simulink model "B_SISO_Simulink"  (R2019a)
settings: Solver=VariableStepAuto  StartTime=0.0  StopTime=50  RelTol=1e-3
values from neighbouring files (symbols this model uses):
  A = [yv (yp+aa0) (yr - 1) (g*cos(tt0)/u0); l_lv l_lp l_lr 0; n_lv n_lp n_lr 0; 0 1 tan(tt0) 0]    [A_Anel_Aberto.m]    (also in B_SISO.m; C_D_LQR_e_Sensores.m = [yv (yp+aa0) (yr - 1) (g*cos(tt0)/u0) 0; l_lv l_lp l_lr 0 0;)
  B = [Yda Ydr ; Lda Ldr ; Nda Ndr ; 0 0]    [A_Anel_Aberto.m]    (also in B_SISO.m; C_D_LQR_e_Sensores.m = [Yda Ydr ; Lda Ldr ; Nda Ndr ; 0 0; 0 0])
  C = [1 0 0 0 ; 0 1 0 0 ; 0 0 1 0 ; 0 0 0 1]    [A_Anel_Aberto.m]    (also in B_SISO.m; C_D_LQR_e_Sensores.m = [1 0 0 0 0; 0 1 0 0 0; 0 0 1 0 0; 0 0 0 1 0; 0 0 0 0 1])
  D = [0 0; 0 0; 0 0; 0 0]    [A_Anel_Aberto.m]    (also in B_SISO.m; C_D_LQR_e_Sensores.m = [0 0; 0 0; 0 0; 0 0; 0 0])
  deg = pi/180    (= 0.0174532777778)    [A_Anel_Aberto.m]    (also in B_SISO.m; C_D_LQR_e_Sensores.m)
  kp = 4.7    [B_SISO.m]
  kr = 1.83    [B_SISO.m]
settings Model: Creator=Antonio Oliveira  LastModifiedBy=Antonio Oliveira

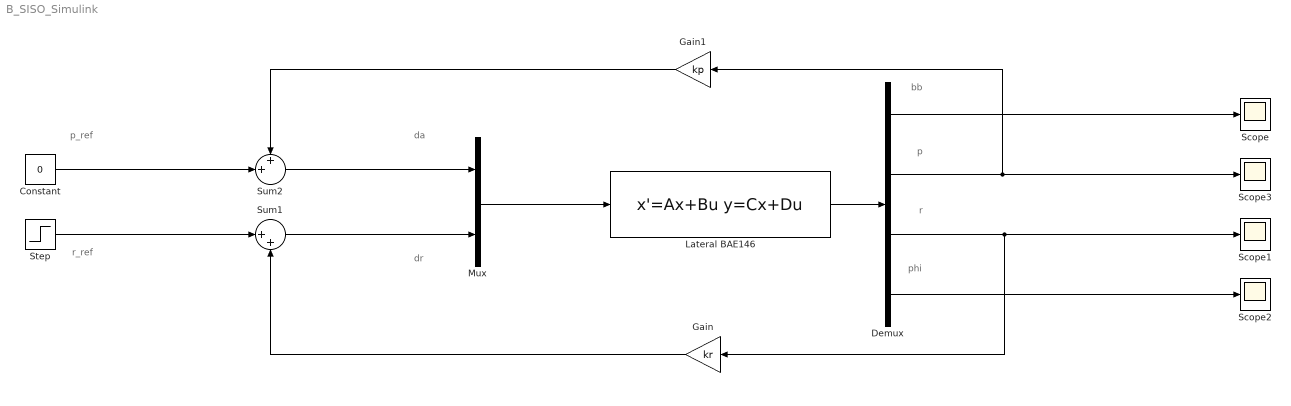
== system B_SISO_Simulink ==
  note: da
  note: bb
  note: p
  note: phi
  note: dr
  note: r
  note: r_ref
  note: p_ref
  Constant : Constant  Value=0
  Demux : Demux
  Gain : Gain  Gain=kr
  Gain1 : Gain  Gain=kp
  "Lateral BAE146 " : StateSpace  A=A  B=B  C=C  D=D  InitialCondition=0  ContinuousStateAttributes='Lateral'
  Mux : Mux  Inputs=2
  Scope{,1..3} (4 alike) : Scope
  Step : Step  Time=0.05  After=20*deg  SampleTime=0  ZeroCross=off
  Sum1 : Sum  Inputs=|++
  Sum2 : Sum  Inputs=++|
  wires:
  Demux/1 -> Scope/1
  Step/1 -> Sum1/1
  Mux/1 -> "Lateral BAE146 "/1
  Sum2/1 -> Mux/1
  Sum1/1 -> Mux/2
  Demux/4 -> Scope2/1
  Gain/1 -> Sum1/2
  Constant/1 -> Sum2/2
  Gain1/1 -> Sum2/1
  "Lateral BAE146 "/1 -> Demux/1
  Demux/2 -> Scope3/1, Gain1/1
  Demux/3 -> Gain/1, Scope1/1
